simulink model "Motion_acc03"  (Simulink 9.0)
settings: Solver=ode1  StartTime=0.0  StopTime=6  FixedStep=h  MaxStep=.1  RelTol=1e-6  AbsTol=1e-8  EnableMultiTasking=on
values from neighbouring files (symbols this model uses):
  b0 = 40    [tuning.m]
  kd = -2.*wc    (= -300)    [tuning.m]
  kp = wc^2    (= 22500)    [tuning.m]
  wo = 40    [tuning.m]
libraries: simulink x2
settings Model: Creator=KingBoy  LastModifiedBy=KingBoy  ExtModeTrigMode=oneshot  ExtModeArmWhenConnect=off
settings DataIOCC: SignalLoggingSaveFormat=ModelDataLogs  SaveOutput=off  TimeSaveName=t  SignalLoggingName=sigsOut
settings OptimizationCC: BooleanDataType=off  LifeSpan=auto
settings DebuggingCC: SaveWithParameterizedLinksMsg=none  SignalResolutionControl=TryResolveAllWithWarning  MultiTaskDSMMsg=warning  MultiTaskCondExecSysMsg=none  SFUnexpectedBacktrackingDiag=error  SFNoUnconditionalDefaultTransitionDiag=error  SFExecutionAtInitializationDiag=warning
settings HardwareCC: TargetUnknown=on
settings CodeAppCC: StateflowObjectComments=off
settings GRTTargetCC: CombineOutputUpdateFcns=off  GRTInterface=on

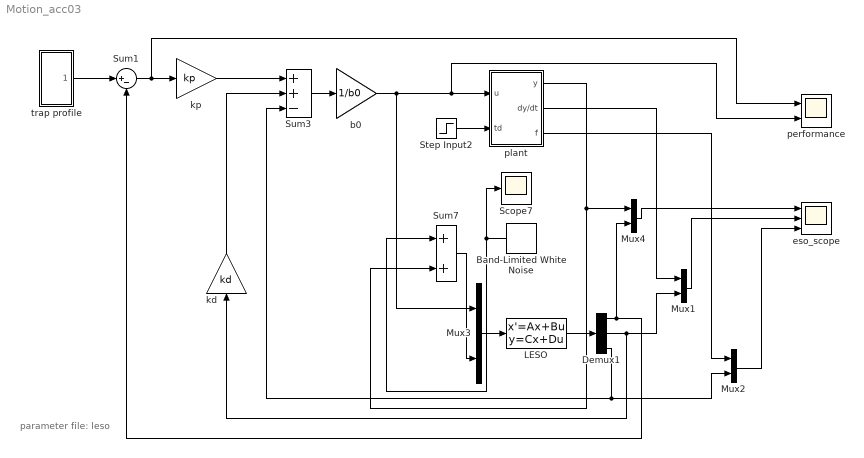
== system Motion_acc03 ==
  note: parameter file: leso
  Band-Limited White Noise : simulink/Sources/Band-Limited White Noise  Cov=[1e-9]  Ts=0.001  seed=[23341]
  Demux1 : Demux  Outputs=3
  "LESO " : StateSpace  A=[-3*wo 1 0;-3*wo^2 0 1; -wo^3 0 0]  B=[0 3*wo ;b0 3*wo^2 ; 0 wo^3 ]  C=eye(3)  D=[0,0;0,0;0,0]  InitialCondition=0
  Mux{1..4} (4 alike) : Mux  Inputs=2
  Scope7 : Scope
  Step Input2 : Step  Time=2  After=-1.16
  Sum1 : Sum  Inputs=|+-  SaturateOnIntegerOverflow=on  InputSameDT=on  OutDataTypeStr=Inherit: Same as first input
  Sum3 : Sum  Inputs=++-  SaturateOnIntegerOverflow=on  InputSameDT=on  OutDataTypeStr=Inherit: Same as first input
  Sum7 : Sum  SaturateOnIntegerOverflow=on  InputSameDT=on  OutDataTypeStr=Inherit: Same as first input
  b0 : Gain  Gain=1/b0  SaturateOnIntegerOverflow=on  OutDataTypeStr=Inherit: Same as input  ParamDataTypeStr=Inherit: Same as input
  eso_scope : Scope  NumInputPorts=3
  kd : Gain  Gain=kd  SaturateOnIntegerOverflow=on  OutDataTypeStr=Inherit: Same as input  ParamDataTypeStr=Inherit: Same as input
  kp : Gain  Gain=kp  SaturateOnIntegerOverflow=on  OutDataTypeStr=Inherit: Same as input  ParamDataTypeStr=Inherit: Same as input
  performance : Scope  NumInputPorts=2
  plant : Subsystem
  trap profile : Subsystem
  wires:
  kp/1 -> Sum3/1
  kd/1 -> Sum3/2
  trap profile/1(Out1) -> Sum1/1
  plant/1("y ") -> Sum7/2, Mux4/1
  b0/1 -> plant/1(u), performance/2, Mux3/1
  Step Input2/1 -> plant/2(td)
  Mux3/1 -> "LESO "/1
  Demux1/3 -> Sum3/3, Mux2/2
  Demux1/2 -> kd/1, Mux1/2
  Demux1/1 -> Sum1/2, Mux4/2
  "LESO "/1 -> Demux1/1
  Sum7/1 -> Mux3/2
  Band-Limited White Noise/1 -> Sum7/1, Scope7/1
  Sum3/1 -> b0/1
  Mux4/1 -> eso_scope/1
  Sum1/1 -> kp/1, performance/1
  Mux1/1 -> eso_scope/2
  plant/2(dy/dt) -> Mux1/1
  Mux2/1 -> eso_scope/3
  plant/3(f) -> Mux2/1

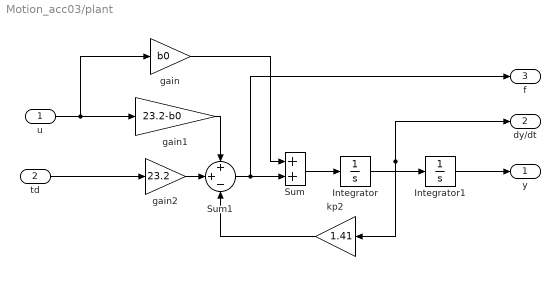
== system Motion_acc03/plant ==
  u : Inport
  td : Inport  Port=2
  Integrator : Integrator
  Integrator1 : Integrator
  Sum : Sum  SaturateOnIntegerOverflow=on  InputSameDT=on  OutDataTypeStr=Inherit: Same as first input
  Sum1 : Sum  Inputs=++-  SaturateOnIntegerOverflow=on  InputSameDT=on  OutDataTypeStr=Inherit: Same as first input
  gain : Gain  Gain=b0  SaturateOnIntegerOverflow=on  OutDataTypeStr=Inherit: Same as input  ParamDataTypeStr=Inherit: Same as input
  gain1 : Gain  Gain=23.2-b0  SaturateOnIntegerOverflow=on  OutDataTypeStr=Inherit: Same as input  ParamDataTypeStr=Inherit: Same as input
  gain2 : Gain  Gain=23.2  SaturateOnIntegerOverflow=on  OutDataTypeStr=Inherit: Same as input  ParamDataTypeStr=Inherit: Same as input
  kp2 : Gain  Gain=1.41  SaturateOnIntegerOverflow=on  OutDataTypeStr=Inherit: Same as input  ParamDataTypeStr=Inherit: Same as input
  "y " : Outport
  dy/dt : Outport  Port=2
  f : Outport  Port=3
  wires:
  Integrator/1 -> Integrator1/1, kp2/1, dy/dt/1
  Sum/1 -> Integrator/1
  kp2/1 -> Sum1/3
  gain1/1 -> Sum1/1
  gain2/1 -> Sum1/2
  td/1 -> gain2/1
  gain/1 -> Sum/1
  u/1 -> gain1/1, gain/1
  Sum1/1 -> Sum/2, f/1
  Integrator1/1 -> "y "/1

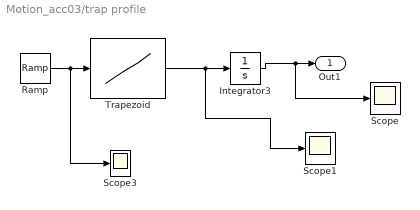
== system Motion_acc03/trap profile ==
  Integrator3 : Integrator  LimitOutput=on  UpperSaturationLimit=10  LowerSaturationLimit=0
  Ramp : simulink/Sources/Ramp  slope=1  start=0  X0=0
  Scope : Scope
  Scope1 : Scope
  Scope3 : Scope
  Trapezoid : Lookup  InputValues=[0 .333333333 .66666666667 1 2]  Table=[0 1.5 1.5 0 0]  SaturateOnIntegerOverflow=on
  Out1 : Outport
  wires:
  Trapezoid/1 -> Integrator3/1, Scope1/1
  Ramp/1 -> Scope3/1, Trapezoid/1
  Integrator3/1 -> Out1/1, Scope/1
